simulink model "GalvoModel_v3_SIMO"  (R2013a)
settings: Solver=ode45  StartTime=0.0  StopTime=10.0  RelTol=1e-3
undefined symbols (not defined in the file or in its folder): BEM, CL, CR, FR, KTR, RIN, TRC
settings Model: Creator=mainster  LastModifiedBy=mainster
settings DebuggingCC: SolverPrmCheckMsg=none

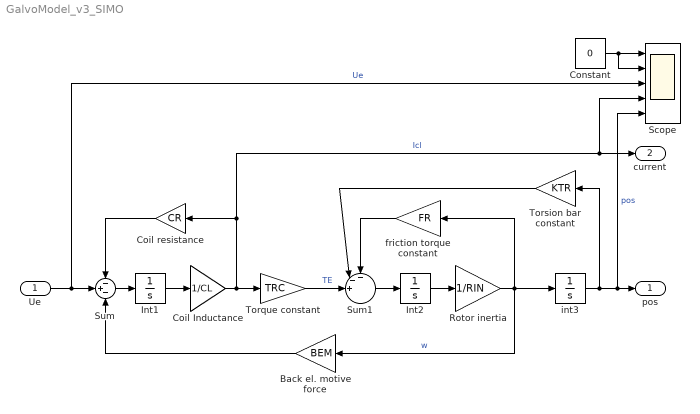
== system GalvoModel_v3_SIMO ==
  Ue : Inport
  Back el. motive force : Gain  Gain=BEM
  Coil Inductance : Gain  Gain=1/CL
  Coil resistance : Gain  Gain=CR
  Constant : Constant  Value=0
  Int1 : Integrator
  Int2 : Integrator
  Rotor inertia : Gain  Gain=1/RIN
  Scope : Scope  NumInputPorts=5
      settings: ShowLegends=on  TimeRange=1.5  YMin=20~0~0~0~0.4  YMax=60~0.002~12~3~1  MaxDataPoints=500000
  Sum : Sum  Inputs=-+-
  Sum1 : Sum  Inputs=--+||
  Torque constant : Gain  Gain=TRC
  Torsion bar constant : Gain  Gain=KTR
  friction torque constant : Gain  Gain=FR
  int3 : Integrator
  pos : Outport
  current : Outport  Port=2
  wires:
  Sum/1 -> Int1/1
  Rotor inertia/1 -> Back el. motive force/1, int3/1, friction torque constant/1  "w"
  int3/1 -> Torsion bar constant/1, Scope/5, pos/1  "pos"
  Int1/1 -> Coil Inductance/1
  Coil Inductance/1 -> Scope/4, current/1, Coil resistance/1, Torque constant/1  "Icl"
  Coil resistance/1 -> Sum/1
  Back el. motive force/1 -> Sum/3
  Int2/1 -> Rotor inertia/1
  friction torque constant/1 -> Sum1/1
  Torsion bar constant/1 -> Sum1/2
  Torque constant/1 -> Sum1/3  "TE"
  Sum1/1 -> Int2/1
  Ue/1 -> Scope/3, Sum/2  "Ue"
  Constant/1 -> Scope/2, Scope/1
